simulink model "Val_trayctoria_d"  (Simulink 7.1)
settings: Solver=ode4  StartTime=0.0  StopTime=6  FixedStep=0.01  RelTol=1e-3
undefined symbols (not defined in the file or in its folder): cdirMitsu, CinDifDir, cinvMitsu, Dterminante, MitsuDin, pol5Grx, pol5Gry, pol5Grz, secuenciax, secuenciay, secuenciaz, Tao_Mitsu
libraries: simulink x3
settings Model: Creator=Dario  LastModifiedBy=Dario

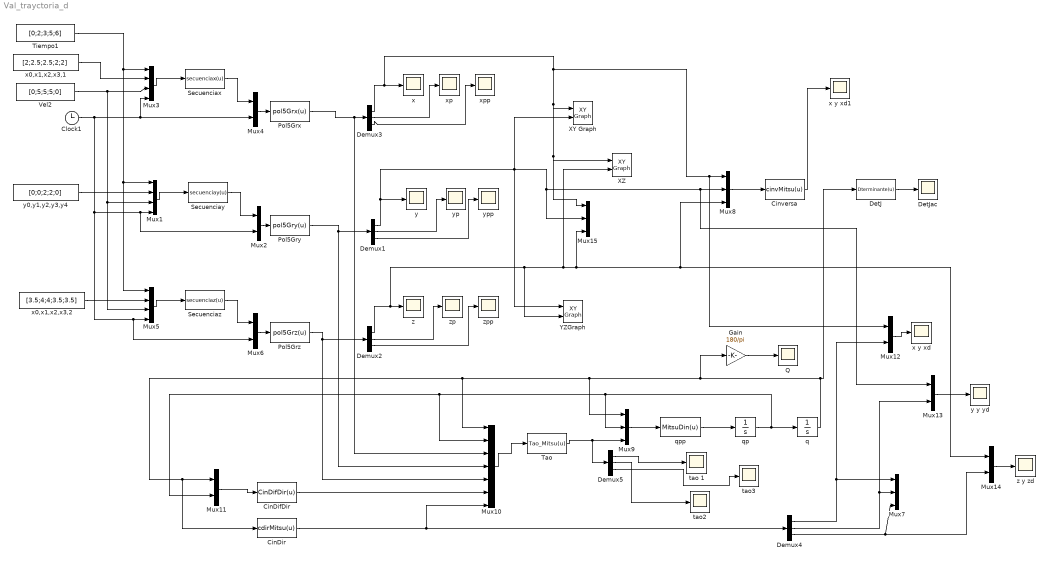
== system Val_trayctoria_d ==
  CinDifDir : MATLABFcn  MATLABFcn=CinDifDir(u)  OutputDimensions=3
  CinDir : MATLABFcn  MATLABFcn=cdirMitsu(u)  OutputDimensions=3
  Cinversa : MATLABFcn  MATLABFcn=cinvMitsu(u)  OutputDimensions=3
  Clock1 : Clock
      settings: Decimation=10
  Demux{1..5} (5 alike) : Demux  Outputs=3
  DetJ : MATLABFcn  MATLABFcn=Dterminante(u)  OutputDimensions=1
  DetJac : Scope
      settings: YMin=9.47975  YMax=9.47982  SaveName=ScopeData6
  Gain : Gain  Gain=180/pi  ParameterDataType=sfix(16)  ParameterScaling=2^0  OutDataType=sfix(16)  OutScaling=2^0
  Mux1 : Mux
  Mux10 : Mux  Inputs=7
  Mux{2,4,6,11..14} (7 alike) : Mux  Inputs=2
  Mux{7..9,15} (4 alike) : Mux  Inputs=3
  Mux3 : Mux
  Mux5 : Mux
  Pol5Grx : MATLABFcn  MATLABFcn=pol5Grx(u)  OutputDimensions=3
  Pol5Gry : MATLABFcn  MATLABFcn=pol5Gry(u)  OutputDimensions=3
  Pol5Grz : MATLABFcn  MATLABFcn=pol5Grz(u)  OutputDimensions=3
  Q : Scope
      settings: YMin=-0.025  YMax=0.3  SaveName=ScopeData16
  Secuenciax : MATLABFcn  MATLABFcn=secuenciax(u)  OutputDimensions=6
  Secuenciay : MATLABFcn  MATLABFcn=secuenciay(u)  OutputDimensions=6
  Secuenciaz : MATLABFcn  MATLABFcn=secuenciaz(u)  OutputDimensions=6
  Tao : MATLABFcn  MATLABFcn=Tao_Mitsu(u)  OutputDimensions=3
  Tiempo1 : Constant  Value=[0;2;3;5;6]  OutDataType=sfix(16)  OutScaling=2^0
  Vel2 : Constant  Value=[0;5;5;5;0]  OutDataType=sfix(16)  OutScaling=2^0
  XY Graph : simulink/Sinks/XY Graph  SystemSampleTime=-1  xmin=-10  xmax=10  ymin=-10  ymax=10  st=-1
  XZ : simulink/Sinks/XY Graph  SystemSampleTime=-1  xmin=-10  xmax=10  ymin=-10  ymax=10  st=-1
  YZGraph : simulink/Sinks/XY Graph  SystemSampleTime=-1  xmin=-10  xmax=10  ymin=-10  ymax=10  st=-1
  q : Integrator
  qp : Integrator
  qpp : MATLABFcn  MATLABFcn=MitsuDin(u)  OutputDimensions=3
  tao 1 : Scope
      settings: SaveName=ScopeData13
  tao2 : Scope
      settings: SaveName=ScopeData14
  tao3 : Scope
      settings: YMin=-17  YMax=6  SaveName=ScopeData15
  x : Scope
      settings: SaveName=ScopeData7
  x y xd : Scope
      settings: YMin=0.95  YMax=2.1  SaveName=ScopeData10
  x y xd1 : Scope
      settings: YMin=0.95  YMax=2.1  SaveName=ScopeData17
  x0,x1,x2,x3,1 : Constant  Value=[2;2.5;2.5;2;2]  OutDataType=sfix(16)  OutScaling=2^0
  x0,x1,x2,x3,2 : Constant  Value=[3.5;4;4;3.5;3.5]  OutDataType=sfix(16)  OutScaling=2^0
  xp : Scope
      settings: SaveName=ScopeData8
  xpp : Scope
      settings: SaveName=ScopeData9
  y : Scope
  y y yd : Scope
      settings: YMin=-0.03  YMax=0.15  SaveName=ScopeData11
  y0,y1,y2,y3,y4 : Constant  Value=[0;0;2;2;0]  OutDataType=sfix(16)  OutScaling=2^0
  yp : Scope
  ypp : Scope
      settings: SaveName=ScopeData2
  z : Scope
      settings: SaveName=ScopeData3
  z y zd : Scope
      settings: YMin=3.5  YMax=5.8  SaveName=ScopeData12
  zp : Scope
      settings: SaveName=ScopeData4
  zpp : Scope
      settings: SaveName=ScopeData5
  wires:
  Mux3/1 -> Secuenciax/1
  Tiempo1/1 -> Mux3/1, Mux1/1, Mux5/1
  x0,x1,x2,x3,1/1 -> Mux3/2
  Clock1/1 -> Mux3/4, Mux4/2, Mux1/4, Mux2/2, Mux5/4, Mux6/2
  Mux4/1 -> Pol5Grx/1
  Vel2/1 -> Mux3/3, Mux1/3, Mux5/3
  Secuenciax/1 -> Mux4/1
  Pol5Grx/1 -> Demux3/1, Mux10/3
  Demux3/1 -> x/1, XY Graph/1, XZ/1, Mux15/1, Mux8/1, Mux12/1
  Demux3/2 -> xp/1
  Demux3/3 -> xpp/1
  Mux1/1 -> Secuenciay/1
  y0,y1,y2,y3,y4/1 -> Mux1/2
  Mux2/1 -> Pol5Gry/1
  Secuenciay/1 -> Mux2/1
  Pol5Gry/1 -> Demux1/1, Mux10/4
  Demux1/1 -> y/1, XY Graph/2, YZGraph/1, Mux8/2, Mux13/1, Mux15/2
  Demux1/2 -> yp/1
  Demux1/3 -> ypp/1
  Mux5/1 -> Secuenciaz/1
  x0,x1,x2,x3,2/1 -> Mux5/2
  Mux6/1 -> Pol5Grz/1
  Secuenciaz/1 -> Mux6/1
  Pol5Grz/1 -> Demux2/1, Mux10/5
  Demux2/1 -> z/1, YZGraph/2, XZ/2, Mux8/3, Mux14/1, Mux15/3
  Demux2/2 -> zp/1
  Demux2/3 -> zpp/1
  Mux8/1 -> Cinversa/1
  DetJ/1 -> DetJac/1
  qpp/1 -> qp/1
  qp/1 -> q/1, Mux9/2, Mux10/2, Mux11/2
  Mux9/1 -> qpp/1
  Tao/1 -> Mux9/3, Demux5/1
  Mux10/1 -> Tao/1
  CinDifDir/1 -> Mux10/6
  Mux11/1 -> CinDifDir/1
  CinDir/1 -> Demux4/1, Mux10/7
  Mux12/1 -> x y xd/1
  Demux4/1 -> Mux12/2, Mux7/1
  Demux4/2 -> Mux13/2, Mux7/2
  Demux4/3 -> Mux14/2, Mux7/3
  Mux13/1 -> y y yd/1
  Mux14/1 -> z y zd/1
  Demux5/1 -> tao 1/1
  Demux5/2 -> tao2/1
  Demux5/3 -> tao3/1
  q/1 -> Mux9/1, Mux10/1, Mux11/1, CinDir/1, Gain/1, DetJ/1
  Gain/1 -> Q/1
  Cinversa/1 -> x y xd1/1
